simulink model "FiltrosDigitais"  (R2018a)
settings: Solver=FixedStepDiscrete  StartTime=0.0  StopTime=0.1  FixedStep=50e-6  RelTol=1e-3
undefined symbols (not defined in the file or in its folder): b, Ts
libraries: dspfdesign x1
settings Model: Creator=daniemot  LastModifiedBy=daniemot

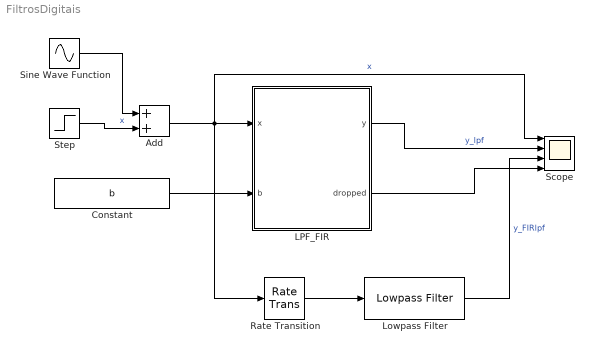
== system FiltrosDigitais ==
  Add : Sum
  Constant : Constant  Value=b
  LPF_FIR : MATLAB Function  TreatAsAtomicUnit=on  SystemSampleTime=Ts
  Lowpass Filter : dspfdesign/Lowpass Filter  FilterType=FIR  DesignForMinimumOrder=on  FilterOrder=50  PassbandFrequency=70  StopbandFrequency=90  PassbandRipple=0.1  StopbandAttenuation=80  InheritSampleRate=off  SampleRate=20000  SimulateUsing=Interpreted execution  roundingMode=Floor  coeffsDataTypeStr=fixdt(1,16)
  Rate Transition : RateTransition  OutPortSampleTime=Ts
  Scope : Scope  NumInputPorts=4
  Sine Wave Function : Sin  Frequency=2*pi*100  SampleTime=0
  Step : Step  Time=100000  After=2  SampleTime=0
  wires:
  Add/1 -> Rate Transition/1, LPF_FIR/1(x), Scope/1  "x"
  Constant/1 -> LPF_FIR/2(b)
  Step/1 -> Add/2  "x"
  Sine Wave Function/1 -> Add/1
  LPF_FIR/1(y) -> Scope/2  "y_lpf"
  LPF_FIR/2(dropped) -> Scope/4
  Lowpass Filter/1 -> Scope/3  "y_FIRlpf"
  Rate Transition/1 -> Lowpass Filter/1

== matlab function FiltrosDigitais/LPF_FIR ==
  data: x input; y output; b input; dropped output
%%%%%%%%%%%%%%%%%%%%%%%%%%%%%%%%%%%%%%%%%%%%%%%%%%%%%%%%%%%%%%%%%%%%%%%%%%
% LPF FIR max 51
%%%%%%%%%%%%%%%%%%%%%%%%%%%%%%%%%%%%%%%%%%%%%%%%%%%%%%%%%%%%%%%%%%%%%%%%%%
% Prog/rev history
%   Mota - 2021-04-19: first release
%
function [y,dropped]   = LPF_FIR ( x, b)

persistent ent N

%%%%%%%%%%%%%%%%%%%%%%%%%%%%%%%%%%
% Values at the first cycle
%%%%%%%%%%%%%%%%%%%%%%%%%%%%%%%%%%
if isempty(ent)
    N = length(b);
    ent = zeros(1,N);
end
%%%%%%%%%%%%%%%%%%%%%%%%%%%%%%%%%%
% Here the function starts actually
%%%%%%%%%%%%%%%%%%%%%%%%%%%%%%%%%%

dropped = ent(N);

%Updates input vector
for aux = N:-1:2
    ent(aux) = ent(aux-1);
end
ent(1) = x;

%dot product and output
y = dot(b, ent);
